simulink model "rot5"  (R2015a)
settings: Solver=ode45  StartTime=0.0  StopTime=10.0  RelTol=1e-3
undefined symbols (not defined in the file): R, theta_ref, Ts, x_ref, y_ref
settings Model: CovSFcnEnable=off  Creator=sebastian  LastModifiedBy=Alexander
settings DebuggingCC: SolverPrmCheckMsg=warning

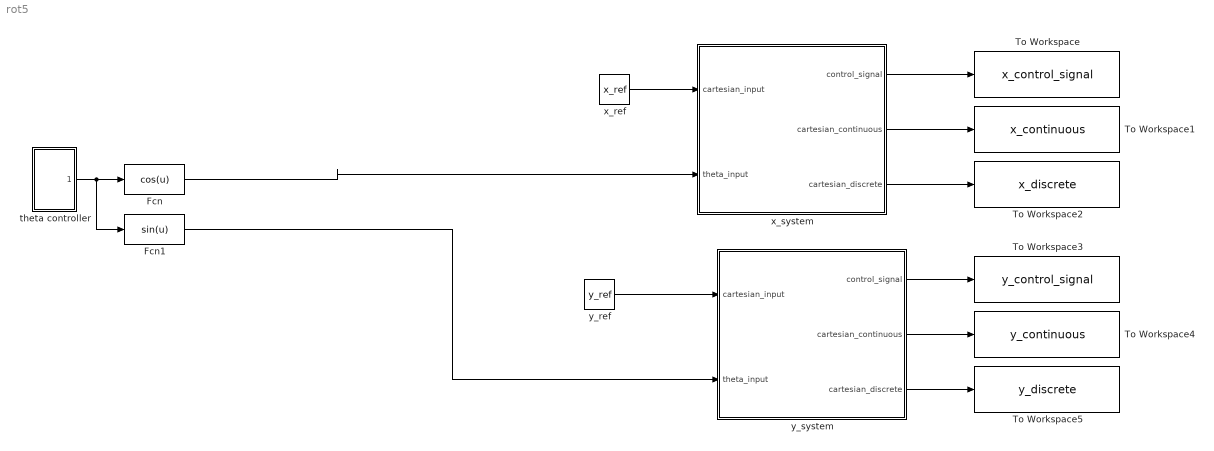
== system rot5 ==
  Fcn : Fcn  Expr=cos(u)
  Fcn1 : Fcn  Expr=sin(u)
  To Workspace : ToWorkspace  VariableName=x_control_signal  SaveFormat=Timeseries  SampleTime=-1
  To Workspace1 : ToWorkspace  VariableName=x_continuous  SaveFormat=Timeseries  SampleTime=-1
  To Workspace2 : ToWorkspace  VariableName=x_discrete  SaveFormat=Timeseries  SampleTime=-1
  To Workspace3 : ToWorkspace  VariableName=y_control_signal  SaveFormat=Timeseries  SampleTime=-1
  To Workspace4 : ToWorkspace  VariableName=y_continuous  SaveFormat=Timeseries  SampleTime=-1
  To Workspace5 : ToWorkspace  VariableName=y_discrete  SaveFormat=Timeseries  SampleTime=-1
  theta controller : Subsystem
  x_ref : Constant  Value=x_ref
  x_system : Subsystem
  y_ref : Constant  Value=y_ref
  y_system : Subsystem
  wires:
  theta controller/1(theta_k) -> Fcn1/1, Fcn/1
  x_ref/1 -> x_system/1(cartesian_input)
  Fcn/1 -> x_system/2(theta_input)
  x_system/1(control_signal) -> To Workspace/1
  x_system/2(cartesian_continuous) -> To Workspace1/1
  x_system/3(cartesian_discrete) -> To Workspace2/1
  y_system/1(control_signal) -> To Workspace3/1
  y_system/2(cartesian_continuous) -> To Workspace4/1
  y_system/3(cartesian_discrete) -> To Workspace5/1
  Fcn1/1 -> y_system/2(theta_input)
  y_ref/1 -> y_system/1(cartesian_input)

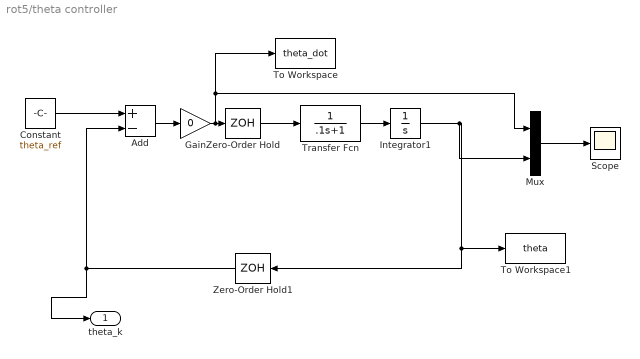
== system rot5/theta controller ==
  Add : Sum  Inputs=+-
  Constant : Constant  Value=theta_ref
  Gain : Gain  Gain=0
  Integrator1 : Integrator  InitialCondition=1
  Mux : Mux  Inputs=2
  Scope : Scope
  To Workspace : ToWorkspace  VariableName=theta_dot  SaveFormat=Timeseries  SampleTime=-1
  To Workspace1 : ToWorkspace  VariableName=theta  SaveFormat=Timeseries  SampleTime=-1
  Transfer Fcn : TransferFcn  Denominator=[.1 1]
  Zero-Order Hold : ZeroOrderHold  SampleTime=Ts
  Zero-Order Hold1 : ZeroOrderHold  SampleTime=Ts
  theta_k : Outport
  wires:
  Constant/1 -> Add/1
  Zero-Order Hold/1 -> Transfer Fcn/1
  Gain/1 -> To Workspace/1, Mux/1, Zero-Order Hold/1
  Zero-Order Hold1/1 -> Add/2, theta_k/1
  Transfer Fcn/1 -> Integrator1/1
  Integrator1/1 -> Mux/2, Zero-Order Hold1/1, To Workspace1/1
  Add/1 -> Gain/1
  Mux/1 -> Scope/1

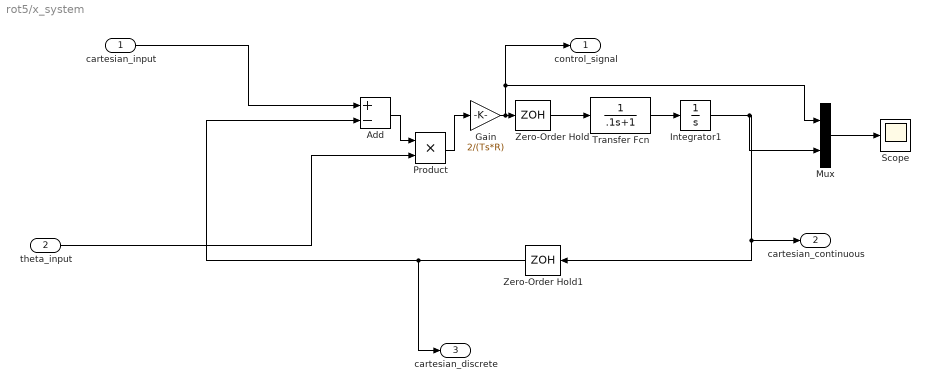
== system rot5/x_system ==
  cartesian_input : Inport
  theta_input : Inport  Port=2
  Add : Sum  Inputs=+-
  Gain : Gain  Gain=2/(Ts*R)
  Integrator1 : Integrator  InitialCondition=1
  Mux : Mux  Inputs=2
  Product : Product
  Scope : Scope
  Transfer Fcn : TransferFcn  Denominator=[.1 1]
  Zero-Order Hold : ZeroOrderHold  SampleTime=Ts
  Zero-Order Hold1 : ZeroOrderHold  SampleTime=Ts
  control_signal : Outport
  cartesian_continuous : Outport  Port=2
  cartesian_discrete : Outport  Port=3
  wires:
  Zero-Order Hold1/1 -> cartesian_discrete/1, Add/2
  Gain/1 -> control_signal/1, Mux/1, Zero-Order Hold/1
  Mux/1 -> Scope/1
  Transfer Fcn/1 -> Integrator1/1
  cartesian_input/1 -> Add/1
  Zero-Order Hold/1 -> Transfer Fcn/1
  Integrator1/1 -> Mux/2, cartesian_continuous/1, Zero-Order Hold1/1
  Product/1 -> Gain/1
  theta_input/1 -> Product/2
  Add/1 -> Product/1

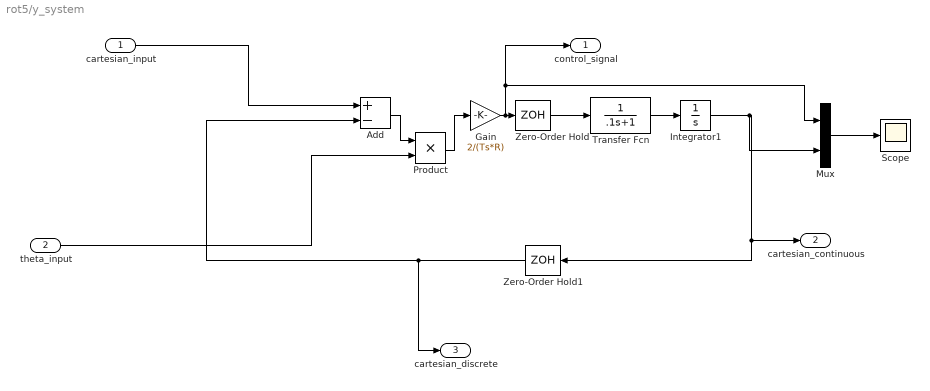
== system rot5/y_system ==
  cartesian_input : Inport
  theta_input : Inport  Port=2
  Add : Sum  Inputs=+-
  Gain : Gain  Gain=2/(Ts*R)
  Integrator1 : Integrator  InitialCondition=1
  Mux : Mux  Inputs=2
  Product : Product
  Scope : Scope
  Transfer Fcn : TransferFcn  Denominator=[.1 1]
  Zero-Order Hold : ZeroOrderHold  SampleTime=Ts
  Zero-Order Hold1 : ZeroOrderHold  SampleTime=Ts
  control_signal : Outport
  cartesian_continuous : Outport  Port=2
  cartesian_discrete : Outport  Port=3
  wires:
  Zero-Order Hold1/1 -> cartesian_discrete/1, Add/2
  Gain/1 -> control_signal/1, Mux/1, Zero-Order Hold/1
  Mux/1 -> Scope/1
  Transfer Fcn/1 -> Integrator1/1
  cartesian_input/1 -> Add/1
  Zero-Order Hold/1 -> Transfer Fcn/1
  Integrator1/1 -> Mux/2, cartesian_continuous/1, Zero-Order Hold1/1
  Product/1 -> Gain/1
  theta_input/1 -> Product/2
  Add/1 -> Product/1
